simulink model "Aufgabe3"  (R2015b)
settings: Solver=VariableStepAuto  StartTime=0.0  StopTime=0.005  RelTol=1e-3
InitFcn:
  | Aufgabe3_calc
values from neighbouring files (symbols this model uses):
  R1 = U/ I    (= 10000)    [Aufgabe2_calc.m]    (also in Aufgabe3_calc.m = 0.1)
  R2 = 10E+3    (= 10000)    [Aufgabe3_calc.m]
libraries: fl_lib x10, nesl_utility x5, elec_lib x3
settings Model: Creator=lukaskiechle  LastModifiedBy=lukaskiechle
settings DebuggingCC: MaxConsecutiveZCsMsg=none
settings SimscapeCC: SimscapeLogType=all  SimscapeLogOpenViewer=on

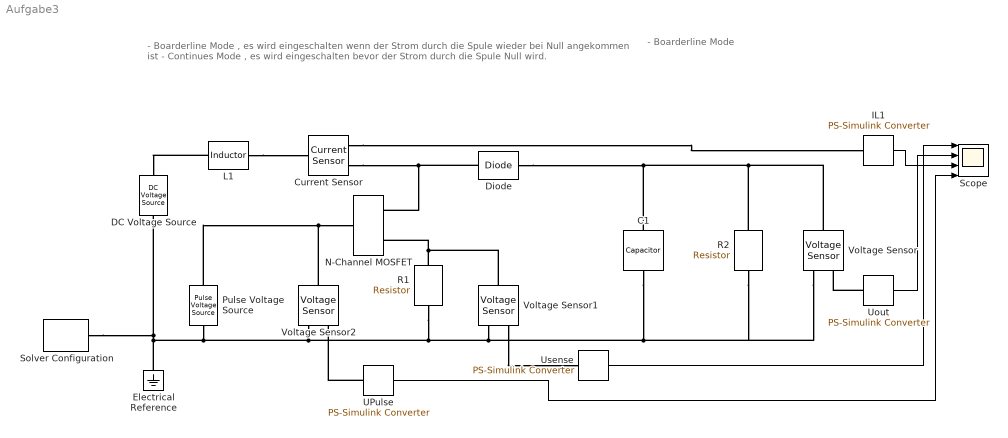
== system Aufgabe3 ==
  note: - Boarderline Mode
  note: - Boarderline Mode , es wird eingeschalten wenn der Strom durch die Spule wieder bei Null angekommen ist
      | - Continues Mode , es wird eingeschalten bevor der Strom durch die Spule Null wird.
  C1 : fl_lib/Electrical/Electrical Elements/Capacitor  c=C1 F  r=1e-6 Ohm  g=0 1/Ohm  i_specify=off  i_priority=None  i=0 A  v_specify=off  v_priority=None  v=0 V  vc_specify=off  vc_priority=None  vc=0 V
  Current Sensor : fl_lib/Electrical/Electrical Sensors/Current Sensor
  DC Voltage Source : fl_lib/Electrical/Electrical Sources/DC Voltage Source  v0=Uin V
  Diode : elec_lib/Semiconductor Devices/Diode  ModelType=2  Vf=0.6 V  Ron=0.1 Ohm  Goff=1e-8 S  Rz=0.1 Ohm  Vz=160 V  C_PWL=5 pF  prmExp=1  I12=[ 0.0137 0.545 ] A  V12=[ 0.6 0.7 ] V  I1=0.0137 A  V1=0.6 V  RS=0.01 Ohm  IS=1e-12 A  Tmeas=25 C  ec=1  BV=Inf V  C_param=1  CJ0=5 pF  VJ=1 V  Mgrad=0.5  Vvec=[ 0.1 10 100 ] V  Cvec=[ 3.5 1 0.4 ] pF  FC=0.5  Q_param=1  Irrm=-7.15 A  iF=4 A  didt=-750 A/us  trr=115 ns  TT=50 ns  tau=100 ns  T_param=1  IS_T2=1.25e-7 A  I1_T2=0.245 A  V1_T2=0.5 V  Tmeas2=125 C  EG_param=1  EG=1.11 eV  XTI_param=1  XTI=3  dBVdT=0 V/K  Tdevice=25 C  Rth=[ 0 10 ] K/W  thermal_mass_parameterization=1  thermal_mass=[ 0 1 ] J/K  thermal_time_constant=[ 0 10 ] s  thermal_mass_initial_temperatures=[ 25 25 ] C
  Electrical Reference : fl_lib/Electrical/Electrical Elements/Electrical Reference
  IL1 : nesl_utility/PS-Simulink Converter  PhysicalDomain=network_engine_domain  SubClassName=ps_output  LeftPortType=input  RightPortType=output  PseudoPeriodic=off  Frequencies=[]  Unit=A  AffineConversion=off
  L1 : fl_lib/Electrical/Electrical Elements/Inductor  l=L1 H  r=0 Ohm  g=1e-9 1/Ohm  i_specify=off  i_priority=None  i=0 A  v_specify=off  v_priority=None  v=0 V  i_L_specify=off  i_L_priority=None  i_L=0 A
  N-Channel MOSFET : elec_lib/Semiconductor Devices/N-Channel MOSFET  parameterization=1  prmDatasheet=1  prmEquCoeff=1  Beta=5 A/V^2  Rds=0.025 Ohm  Id=50 A  Vgs=5 V  Vth=1.7 V  lam=0 1/V  Tmeas=25 C  RS=1e-4 Ohm  RD=0.01 Ohm  C_param=1  C_GS=270 pF  C_GD=80 pF  C_iss=350 pF  C_rss=80 pF  C_oss=0 pF  C_GS_vec=[ 270 300 290 280 295 255 ] pF  C_GD_vec=[ 450 400 300 190 95 55 ] pF  C_iss_vec=[ 720 700 590 470 390 310 ] pF  C_rss_vec=[ 450 400 300 190 95 55 ] pF  C_oss_vec=[ 900 810 690 420 270 170 ] pF  C_Vds_vec=[ 0.1 0.3 1 3 10 30 ] V  charge_linearity_param=1  C_OX=200 pF  V_C_OX=-0.5 V  dVth_dT=-6 mV/K  Rds_T2=0.037 Ohm  Tmeas2=125 C  BEXDatasheet=-1.5  BEXEquCoeff=-1.5  TdeviceDatasheet=25 C  TdeviceEquCoeff=25 C  Rth=[ 0 10 ] K/W  thermal_mass_parameterization=1  thermal_mass=[ 0 1 ] J/K  thermal_time_constant=[ 0 10 ] s  thermal_mass_initial_temperatures=[ 25 25 ] C
  Pulse Voltage Source : elec_lib/Additional Components/SPICE-Compatible Components/Sources/Pulse Voltage Source  V1=0 V  V2=10 V  TD=1e-9 s  TR=1e-9 s  TF=1e-9 s  PW=Ton s  PER=Twidth s
  R1 : fl_lib/Electrical/Electrical Elements/Resistor  R=R1 Ohm  i_specify=off  i_priority=None  i=0 A  v_specify=off  v_priority=None  v=0 V
  R2 : fl_lib/Electrical/Electrical Elements/Resistor  R=R2 Ohm  i_specify=off  i_priority=None  i=0 A  v_specify=off  v_priority=None  v=0 V
  Scope : Scope  NumInputPorts=4
  Solver Configuration : nesl_utility/Solver Configuration  PhysicalDomain=network_engine_domain  SubClassName=solver  LeftPortType=input  RightPortType=generic  Accelerate=off  Tones=[]  Harmonics=[]  SimulateNoise=off  Profile=off  UseLocalSampling=off  EnableSwitchedLinearOptims=on  FrequencyDomain=off  UseCCode=off  RelTol=0.001  AbsTol=1e-06  MinStep=1e-09  ToWorkspace=off  RevertToSquareIcSolve=off  NumHomotopyIterations=100  PhasorMode=off  PhasorModeNumHarmonics=1  DoDC=on  ResidualTolerance=1e-09  UseLocalSolver=off  LocalSolverChoice=NE_BACKWARD_EULER_ADVANCER  LocalSolverSampleTime=0.001  DoFixedCost=off  MaxNonlinIter=3  MaxModeIter=2  LinearAlgebra=Sparse  DelaysMemoryBudget=1024  AutomaticFiltering=on  FilteringTimeConstant=0.001
  UPulse : nesl_utility/PS-Simulink Converter  PhysicalDomain=network_engine_domain  SubClassName=ps_output  LeftPortType=input  RightPortType=output  PseudoPeriodic=off  Frequencies=[]  Unit=V  AffineConversion=off
  Uout : nesl_utility/PS-Simulink Converter  PhysicalDomain=network_engine_domain  SubClassName=ps_output  LeftPortType=input  RightPortType=output  PseudoPeriodic=off  Frequencies=[]  Unit=V  AffineConversion=off
  Usense : nesl_utility/PS-Simulink Converter  PhysicalDomain=network_engine_domain  SubClassName=ps_output  LeftPortType=input  RightPortType=output  PseudoPeriodic=off  Frequencies=[]  Unit=V  AffineConversion=off
  Voltage Sensor : fl_lib/Electrical/Electrical Sensors/Voltage Sensor
  Voltage Sensor1 : fl_lib/Electrical/Electrical Sensors/Voltage Sensor
  Voltage Sensor2 : fl_lib/Electrical/Electrical Sensors/Voltage Sensor
  wires:
  UPulse/1 -> Scope/4
  Usense/1 -> Scope/1
  Uout/1 -> Scope/2
  IL1/1 -> Scope/3
  connections:
  L1/LConn1 -- DC Voltage Source/LConn1
  L1/RConn1 -- Current Sensor/LConn1
  Current Sensor/RConn2 -- Diode/LConn1 -- N-Channel MOSFET/RConn1
  Electrical Reference/LConn1 -- Voltage Sensor2/RConn2 -- R1/RConn1 -- R2/RConn1 -- Voltage Sensor/RConn2 -- C1/RConn1 -- Voltage Sensor1/RConn2 -- Pulse Voltage Source/RConn1 -- Solver Configuration/RConn1 -- DC Voltage Source/RConn1
  Voltage Sensor/LConn1 -- R2/LConn1 -- Diode/RConn1 -- C1/LConn1
  Current Sensor/RConn1 -- IL1/LConn1
  Voltage Sensor1/RConn1 -- Usense/LConn1
  Uout/LConn1 -- Voltage Sensor/RConn1
  Pulse Voltage Source/LConn1 -- N-Channel MOSFET/LConn1 -- Voltage Sensor2/LConn1
  R1/LConn1 -- Voltage Sensor1/LConn1 -- N-Channel MOSFET/RConn2
  UPulse/LConn1 -- Voltage Sensor2/RConn1
